simulink model "ModulacionFinal"  (R2020a)
settings: Solver=VariableStepAuto  StartTime=0.0  StopTime=Tsim  MaxStep=1e-8  RelTol=1e-3
values from neighbouring files (symbols this model uses):
  Amplitud = 1    [Sinc_PSKm.m]
  Att_Volt_Canal = 10^(Att_dB / 20)    [Sinc_PSKm.m]
  b = 0.6    [Sinc_PSKm.m]
  C = 1e-6    (= 1e-06)    [Sinc_PSKm.m]
  Frec_port = 100 * Rb    (= 100000)    [Sinc_PSKm.m]
  Pot_Ruido = 2*eta * Ancho_banda_minimo    [Sinc_PSKm.m]
  R1 = Kp * Kv / (wn^2 * C)    (= 98.7654320988)    [Sinc_PSKm.m]
  R2 = 2 * zita / (wn * C)    (= 53.3333333333)    [Sinc_PSKm.m]
  Rb = 1000    [Sinc_PSKm.m]
  Retraso_Canal = Long_Canal / C_canal+0.5/Frec_port    (= 3.83333333333e-05)    [Sinc_PSKm.m]
  Tb = 1 / Rb    (= 0.001)    [Sinc_PSKm.m]
undefined symbols (not defined in the file or in its folder): Ancho_banda_ruido
libraries: powerlib_meascontrol x3, dspsigops x3, commsynccomp2 x2, dsparch4 x1, simulink x1, dspsnks4 x1
settings Model: SimulationMode=accelerator  Creator=Alejandro  LastModifiedBy=LAURA
settings OptimizationCC: LifeSpan=inf
settings DebuggingCC: SFExecutionAtInitializationDiag=none  ArithmeticOperatorsInVariantConditions=warning
settings SFSimCC: CustomCodeUndefinedFunction=UseInterfaceOnly
settings CodeAppCC: StateflowObjectComments=on
settings SimscapeCC: SimscapeNormalizeSystem=off

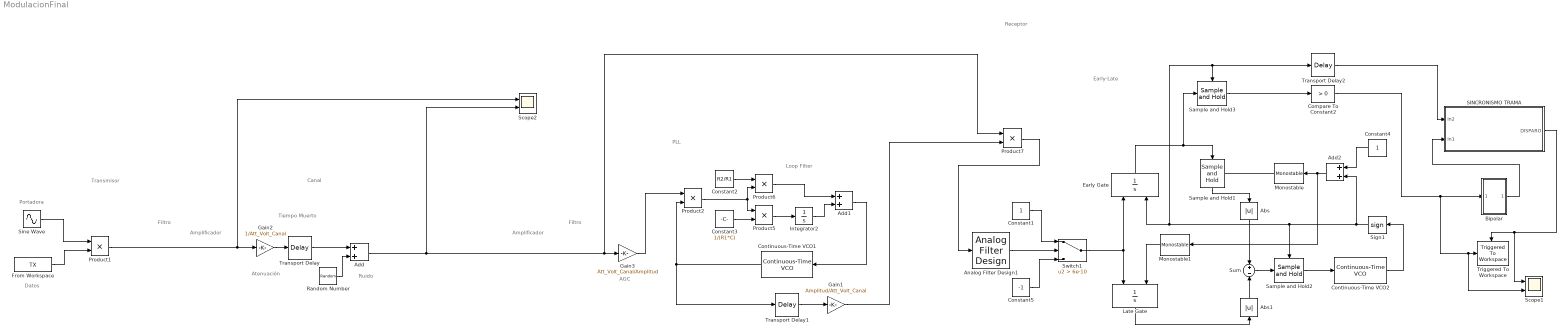
== system ModulacionFinal ==
  note: Receptor
  note: Canal
  note: Ruido
  note: Tiempo Muerto
  note: Atenuación
  note: Amplificador
  note: Filtro
  note: Transmisor
  note: Portadora
  note: Datos
  note: Filtro
  note: Amplificador
  note: PLL
  note: Loop Filter
  note: AGC
  note: Early-Late
  Abs : Abs
  Abs1 : Abs
  Add : Sum
  Add1 : Sum
  Add2 : Sum
  Analog Filter Design1 : dsparch4/Analog Filter Design  method=Butterworth  filttype=Lowpass  N=8  Wlo=2*pi*(Rb)  Whi=80  Rp=2  Rs=40
  "Bipolar " : Subsystem
  Compare To Constant2 : simulink/Logic and Bit Operations/Compare To Constant  relop=>  const=0  OutDataTypeStr=boolean
  Constant1 : Constant
  Constant2 : Constant  Value=R2/R1
  Constant3 : Constant  Value=1/(R1*C)
  Constant4 : Constant
  Constant5 : Constant  Value=-1
  Continuous-Time VCO1 : commsynccomp2/Continuous-Time VCO  Ac=1  Fc=Frec_port  Kc=Kv  Ph=0
      settings: SourceProductBaseCode=CM
  Continuous-Time VCO2 : commsynccomp2/Continuous-Time VCO  Ac=1  Fc=Rb  Kc=kv2  Ph=0
      settings: SourceProductBaseCode=CM
  Early Gate : Integrator  ExternalReset=rising
  From Workspace : FromWorkspace  VariableName=TX  SampleTime=Tb  Interpolate=off  ZeroCross=off  OutputAfterFinalValue=Holding final value
  Gain1 : Gain  Gain=Amplitud/Att_Volt_Canal
  Gain2 : Gain  Gain=1/Att_Volt_Canal
  Gain3 : Gain  Gain=Att_Volt_Canal/Amplitud
  Integrator2 : Integrator
  Late Gate : Integrator  ExternalReset=falling
  Monostable : powerlib_meascontrol/Logic/Monostable  EdgeDetect=Rising  PulseDuration=b*Tb  ic=0  Ts=0
      settings: SourceProductBaseCode=PS
  Monostable1 : powerlib_meascontrol/Logic/Monostable  EdgeDetect=Rising  PulseDuration=(1-b)*Tb  ic=0  Ts=0
      settings: SourceProductBaseCode=PS
  Product{1..2,5..7} (5 alike) : Product
  Random Number : RandomNumber  Variance=Pot_Ruido  SampleTime=0.01/(2*Ancho_banda_ruido)
  "SINCRONISMO TRAMA " : Subsystem
  Sample and Hold1 : dspsigops/Sample and Hold  trig=Falling edge  initCond=0  latchinput=off
  Sample and Hold2 : dspsigops/Sample and Hold  trig=Rising edge  initCond=0  latchinput=off
  Sample and Hold3 : dspsigops/Sample and Hold  trig=Falling edge  initCond=0  latchinput=off
  Scope1 : Scope  NumInputPorts=2
  Scope2 : Scope  NumInputPorts=2
  Sign1 : Signum
  Sine Wave : Sin  Amplitude=Amplitud  Frequency=2*pi*Frec_port  SampleTime=0
  Sum : Sum  Inputs=+|-
  Switch1 : Switch  Criteria=u2 > Threshold  Threshold=6e-10
  Transport Delay : TransportDelay  DelayTime=Retraso_Canal
  Transport Delay1 : TransportDelay  DelayTime=1/(4*Frec_port)
  Transport Delay2 : TransportDelay  DelayTime=113.83e-6
  Triggered To Workspace : dspsnks4/Triggered To Workspace  TriggerType=Rising edge  VariableName=Salida  Buffer=inf  Save2DMode=2-D array (concatenate along first dimension)
      settings: SourceProductBaseCode=DS  FixptAsFi=off
  wires:
  Gain2/1 -> Transport Delay/1
  Product6/1 -> Add1/1
  Integrator2/1 -> Add1/2
  Product5/1 -> Integrator2/1
  Product2/1 -> Product5/1, Product6/2
  Constant3/1 -> Product5/2
  Constant2/1 -> Product6/1
  Add1/1 -> Continuous-Time VCO1/1
  Continuous-Time VCO1/1 -> Transport Delay1/1, Product2/2
  Transport Delay1/1 -> Gain1/1
  Sine Wave/1 -> Product1/1
  Late Gate/1 -> Abs1/1
  Sum/1 -> Sample and Hold2/1
  Sample and Hold2/1 -> Continuous-Time VCO2/1
  Monostable/1 -> Sample and Hold1/Trigger
  Sign1/1 -> Add2/2, Sample and Hold2/Trigger, Early Gate/2, Sample and Hold3/Trigger, Transport Delay2/1
  Abs/1 -> Sum/1
  Monostable1/1 -> Late Gate/2
  Abs1/1 -> Sum/2
  Continuous-Time VCO2/1 -> Sign1/1
  Sample and Hold1/1 -> Abs/1
  Product7/1 -> Analog Filter Design1/1
  Sample and Hold3/1 -> Compare To Constant2/1
  Constant4/1 -> Add2/1
  Add2/1 -> Monostable1/1, Monostable/1
  Gain3/1 -> Product2/1
  Analog Filter Design1/1 -> Switch1/2
  Constant1/1 -> Switch1/1
  Constant5/1 -> Switch1/3
  Switch1/1 -> Early Gate/1, Late Gate/1
  Transport Delay/1 -> Add/1
  Random Number/1 -> Add/2
  Gain1/1 -> Product7/2
  Early Gate/1 -> Sample and Hold1/1, Sample and Hold3/1
  Add/1 -> Scope2/2, Gain3/1, Product7/1
  Product1/1 -> Scope2/1, Gain2/1
  Transport Delay2/1 -> "SINCRONISMO TRAMA "/1(In2)
  "Bipolar "/1(Out1) -> "SINCRONISMO TRAMA "/2(In1)
  Compare To Constant2/1 -> Scope1/2, Triggered To Workspace/1, "Bipolar "/1(In1)
  From Workspace/1 -> Product1/2
  "SINCRONISMO TRAMA "/1("DISPARO ") -> Scope1/1, Triggered To Workspace/Trigger

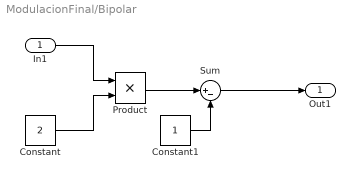
== system ModulacionFinal/Bipolar  ==
  In1 : Inport
  Constant : Constant  Value=2
  Constant1 : Constant
  Product : Product
  Sum : Sum  Inputs=|+-
  Out1 : Outport  VectorParamsAs1DForOutWhenUnconnected=off
  wires:
  Constant1/1 -> Sum/2
  Product/1 -> Sum/1
  Constant/1 -> Product/2
  Sum/1 -> Out1/1
  In1/1 -> Product/1

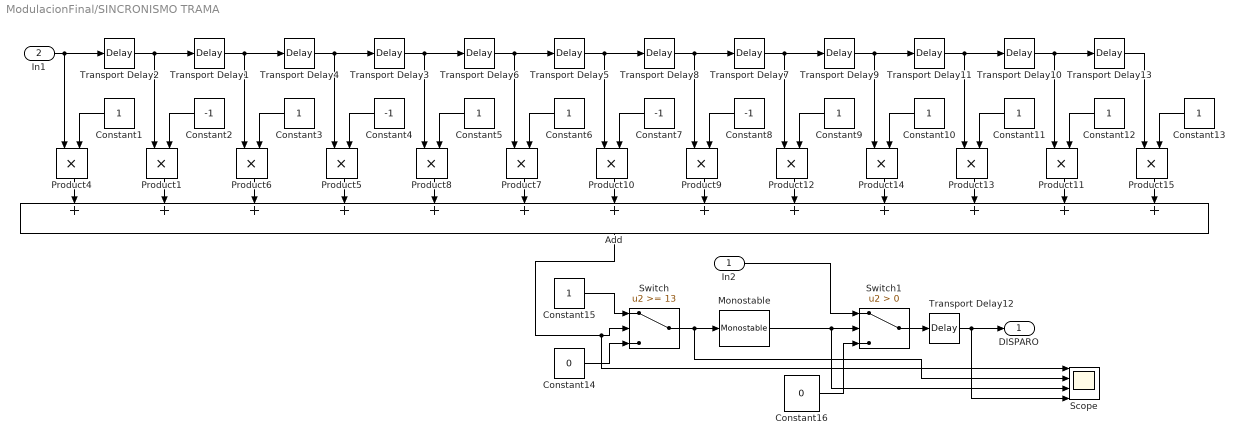
== system ModulacionFinal/SINCRONISMO TRAMA  ==
  In2 : Inport
  In1 : Inport  Port=2
  Add : Sum  Inputs=+++++++++++++
  Constant{1,3,5..6,9..13,15} (10 alike) : Constant
  Constant14 : Constant  Value=0
  Constant16 : Constant  Value=0
  Constant{2,4,7..8} (4 alike) : Constant  Value=-1
  Monostable : powerlib_meascontrol/Logic/Monostable  EdgeDetect=Falling  PulseDuration=Tsim  ic=0  Ts=0
      settings: SourceProductBaseCode=PS
  Product{1,4..15} (13 alike) : Product
  Scope : Scope  NumInputPorts=4
  Switch : Switch  Threshold=13
  Switch1 : Switch  Criteria=u2 > Threshold
  Transport Delay{1..13} (13 alike) : TransportDelay  DelayTime=Tb
  "DISPARO " : Outport  VectorParamsAs1DForOutWhenUnconnected=off
  wires:
  Transport Delay10/1 -> Product11/1, Transport Delay13/1
  Transport Delay1/1 -> Product6/1, Transport Delay4/1
  Add/1 -> Scope/1, Switch/2
  Constant2/1 -> Product1/2
  Product1/1 -> Add/2
  Transport Delay5/1 -> Product10/1, Transport Delay8/1
  Transport Delay11/1 -> Product13/1, Transport Delay10/1
  Product11/1 -> Add/12
  Constant11/1 -> Product13/2
  Transport Delay13/1 -> Product15/1
  Product13/1 -> Add/11
  Transport Delay7/1 -> Product12/1, Transport Delay9/1
  Constant13/1 -> Product15/2
  Constant10/1 -> Product14/2
  Constant9/1 -> Product12/2
  Product14/1 -> Add/10
  Constant12/1 -> Product11/2
  Product12/1 -> Add/9
  Product15/1 -> Add/13
  Product4/1 -> Add/1
  Transport Delay3/1 -> Product8/1, Transport Delay6/1
  Product8/1 -> Add/5
  Product7/1 -> Add/6
  Product9/1 -> Add/8
  Constant5/1 -> Product8/2
  Constant6/1 -> Product7/2
  Transport Delay8/1 -> Product9/1, Transport Delay7/1
  Product10/1 -> Add/7
  Transport Delay6/1 -> Product7/1, Transport Delay5/1
  Constant7/1 -> Product10/2
  Constant8/1 -> Product9/2
  Constant1/1 -> Product4/2
  Transport Delay2/1 -> Product1/1, Transport Delay1/1
  Constant14/1 -> Switch/3
  Product5/1 -> Add/4
  Transport Delay4/1 -> Product5/1, Transport Delay3/1
  Constant3/1 -> Product6/2
  Constant4/1 -> Product5/2
  Product6/1 -> Add/3
  Constant15/1 -> Switch/1
  Transport Delay9/1 -> Product14/1, Transport Delay11/1
  Switch/1 -> Monostable/1, Scope/2
  Constant16/1 -> Switch1/3
  Switch1/1 -> Transport Delay12/1
  In1/1 -> Product4/1, Transport Delay2/1
  In2/1 -> Switch1/1
  Monostable/1 -> Scope/3, Switch1/2
  Transport Delay12/1 -> Scope/4, "DISPARO "/1
